simulink library "cyl2cart"  (R2018b)
settings: Solver=VariableStepAuto  StartTime=0.0  StopTime=10.0  RelTol=1e-3
settings Model: Creator=BI28030  LastModifiedBy=BI28030

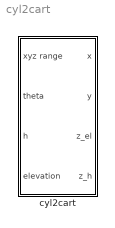
== system cyl2cart ==
  cyl2cart : Subsystem  mask(cyl2cart){}
      mask help: cyl2cart

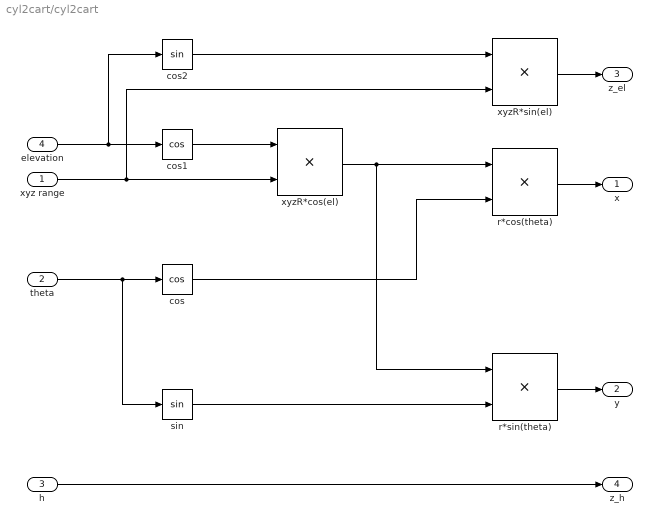
== system cyl2cart/cyl2cart ==
  xyz range : Inport
  theta : Inport  Port=2
  h : Inport  Port=3
  elevation : Inport  Port=4
  cos : Trigonometry  Operator=cos
  cos1 : Trigonometry  Operator=cos
  cos2 : Trigonometry
  r*cos(theta) : Product  RndMeth=Zero
  r*sin(theta) : Product  RndMeth=Zero
  sin : Trigonometry
  xyzR*cos(el) : Product  RndMeth=Zero
  xyzR*sin(el) : Product  RndMeth=Zero
  x : Outport
  y : Outport  Port=2
  z_el : Outport  Port=3
  z_h : Outport  Port=4
  wires:
  r*sin(theta)/1 -> y/1
  sin/1 -> r*sin(theta)/2
  cos/1 -> r*cos(theta)/2
  theta/1 -> cos/1, sin/1
  xyz range/1 -> xyzR*sin(el)/2, xyzR*cos(el)/2
  h/1 -> z_h/1
  r*cos(theta)/1 -> x/1
  elevation/1 -> cos2/1, cos1/1
  cos1/1 -> xyzR*cos(el)/1
  xyzR*cos(el)/1 -> r*cos(theta)/1, r*sin(theta)/1
  cos2/1 -> xyzR*sin(el)/1
  xyzR*sin(el)/1 -> z_el/1
